simulink model "SimulateOpenLoopMultiLevelInverterModel"  (R2018a)
settings: Solver=ode14x  StartTime=0.0  StopTime=10.0  FixedStep=dt  RelTol=1e-3
undefined symbols (not defined in the file or in its folder): I_Idvec, I_Iqvec, IinIC, P_tvec, Vin
libraries: Lib_PB_MultiLevelInverter_TMATS x1
settings Model: Creator=tcarsten  LastModifiedBy=mebell
settings SolverCC: AlgebraicLoopSolver=LineSearch
settings CodeAppCC: StateflowObjectComments=on

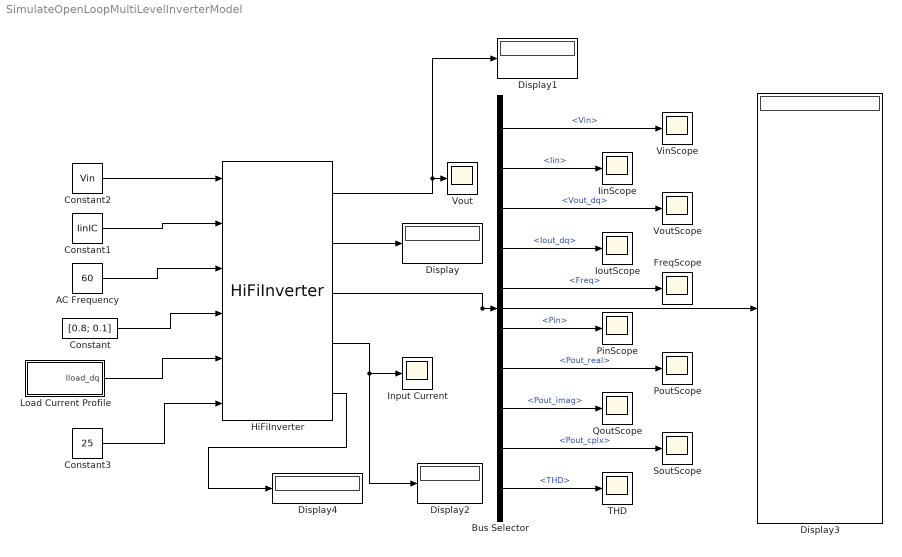
== system SimulateOpenLoopMultiLevelInverterModel ==
  AC Frequency : Constant  Value=60  VectorParams1D=off
  Bus Selector : BusSelector  OutputSignals=Vin,Iin,Vout_dq,Iout_dq,Freq,Pin,Pout_real,Pout_imag,Pout_cplx,THD
  Constant : Constant  Value=[0.8; 0.1]  VectorParams1D=off
  Constant1 : Constant  Value=IinIC  VectorParams1D=off
  Constant2 : Constant  Value=Vin  VectorParams1D=off
  Constant3 : Constant  Value=25
  Display{,1..4} (5 alike) : Display
  FreqScope : Scope
  HiFiInverter : Lib_PB_MultiLevelInverter_TMATS/HiFiInverter  Pdis_M=1  Carm_M=600e-6  Larm_M=0.3e-6  Rarm_M=1.5e-3  NPhases_M=3  NModules_M=401  THD_M=0.10  QgTotal_M=2e-9  Vgate_M=0.5  TRise_M=4e-9  TFall_M=6e-9  Fsw_M=1e6  Trr_M=0  iDesign_copy=2e-9
  IinScope : Scope
  Input Current : Scope
  IoutScope : Scope
  Load Current Profile : Subsystem
  PinScope : Scope
  PoutScope : Scope
  QoutScope : Scope
  SoutScope : Scope
  THD : Scope
  VinScope : Scope
  Vout : Scope
  VoutScope : Scope
  wires:
  Constant2/1 -> HiFiInverter/1
  Bus Selector/3 -> VoutScope/1  "<Vout_dq>"
  Bus Selector/4 -> IoutScope/1  "<Iout_dq>"
  Bus Selector/6 -> PinScope/1  "<Pin>"
  HiFiInverter/3 -> Display3/1, Bus Selector/1
  Bus Selector/7 -> PoutScope/1  "<Pout_real>"
  Bus Selector/8 -> QoutScope/1  "<Pout_imag>"
  HiFiInverter/1 -> Display1/1, Vout/1
  Bus Selector/9 -> SoutScope/1  "<Pout_cplx>"
  Bus Selector/10 -> THD/1  "<THD>"
  AC Frequency/1 -> HiFiInverter/3
  Bus Selector/5 -> FreqScope/1  "<Freq>"
  Bus Selector/2 -> IinScope/1  "<Iin>"
  Bus Selector/1 -> VinScope/1  "<Vin>"
  Constant1/1 -> HiFiInverter/2
  Constant/1 -> HiFiInverter/4
  Load Current Profile/1(Iload_dq) -> HiFiInverter/5
  HiFiInverter/2 -> Display/1
  HiFiInverter/4 -> Input Current/1, Display2/1
  Constant3/1 -> HiFiInverter/6
  HiFiInverter/5 -> Display4/1

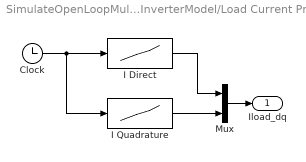
== system SimulateOpenLoopMultiLevelInverterModel/Load Current Profile ==
  Clock : Clock
  I Direct : Lookup_n-D  NumberOfTableDimensions=1  BreakpointsForDimension1=P_tvec  Table=I_Idvec  InternalRulePriority=Speed  RndMeth=Simplest  InputSameDT=on
  I Quadrature : Lookup_n-D  NumberOfTableDimensions=1  BreakpointsForDimension1=P_tvec  Table=I_Iqvec  InternalRulePriority=Speed  RndMeth=Simplest  InputSameDT=on
  Mux : Mux  Inputs=2
  Iload_dq : Outport
  wires:
  Clock/1 -> I Quadrature/1, I Direct/1
  I Quadrature/1 -> Mux/2
  I Direct/1 -> Mux/1
  Mux/1 -> Iload_dq/1
